simulink model "sampleModel7424_pp_difftest"  (R2018a)
settings: Solver=VariableStepAuto  StartTime=0.0  StopTime=10.0  RelTol=1e-3
undefined symbols (not defined in the file): DiscIntNeverNeededParam
libraries: simulink x211
(part 1 of 5)
settings Model: Creator=cyfuzz  LastModifiedBy=shafiul
settings CodeAppCC: StateflowObjectComments=on

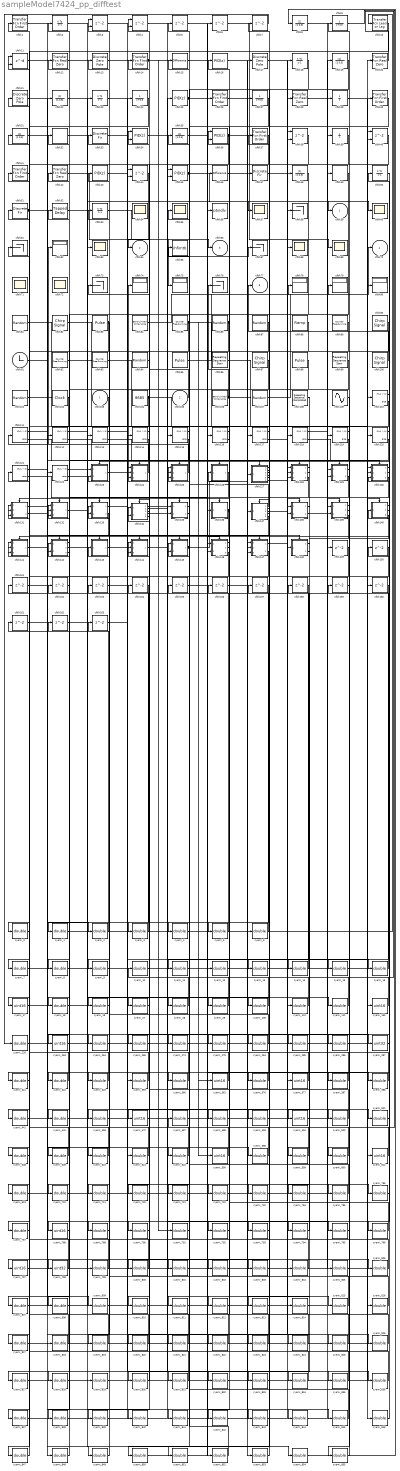
== system sampleModel7424_pp_difftest ==
  cfblk103 : Inport
  cfblk105 : Inport  Port=2
  cfblk{1,14,26,30,37,41} (6 alike) : simulink/Discrete/Transfer Fcn First Order  PoleZ=0.95  ICPrevOutput=0.0  DoSatur=off
      settings: SourceProductName=Simulink
  cfblk10 : simulink/Discrete/Transfer Fcn Lead or Lag  PoleZ=0.95  ZeroZ=0.75  ICPrevOutput=0.0  ICPrevInput=0.0  DoSatur=off
      settings: SourceProductName=Simulink  SourceProductBaseCode=SL
  cfblk{82,90,97,100} (4 alike) : simulink/Sources/Chirp Signal  f1=0.1  T=100  f2=1
  cfblk101 : UniformRandomNumber  SampleTime=0.1
  cfblk102 : DigitalClock
  cfblk104 : Constant  Value=8685  OutDataTypeStr=double  SampleTime=1
  cfblk106 : simulink/Sources/Band-Limited White Noise  Cov=[0.1]  Ts=0.1  seed=[23341]
  cfblk107 : RandomNumber  SampleTime=0.1
  cfblk108 : simulink/Sources/Repeating Sequence Interpolated  OutValues=[3 1 4 2 1].'  TimeValues=[0 0.1 0.5 0.6 1].'  LookUpMeth=Interpolation-Use End Values  tsamp=0.01  OutMin=[]  OutMax=[]  OutDataTypeStr=double  OutputDataTypeScalingMode=double  OutDataType=fixdt(0,8)  OutScaling=2^-10
  cfblk109 : Sin  SampleTime=0
  cfblk11 : Delay  DelayLengthSource=Input port  SampleTime=1
      settings: InputPortMap=u0,p1
  cfblk{110..122} (13 alike) : If  SampleTime=1
  cfblk{12,20,28,42} (4 alike) : simulink/Discrete/Transfer Fcn Real Zero  ZeroZ=0.75  ICPrevInput=0.0  DoSatur=off
      settings: SourceProductName=Simulink  SourceProductBaseCode=SL
  cfblk123 : Subsystem  TreatAsAtomicUnit=on
  cfblk124 : Subsystem  TreatAsAtomicUnit=on
  cfblk125 : Subsystem  TreatAsAtomicUnit=on
  cfblk126 : Subsystem  TreatAsAtomicUnit=on
  cfblk127 : Subsystem  TreatAsAtomicUnit=on
  cfblk128 : Subsystem  TreatAsAtomicUnit=on
  cfblk129 : Subsystem  TreatAsAtomicUnit=on
  cfblk13 : DiscreteZeroPole  Poles=[0 0.5]  Gain=1
  cfblk130 : Subsystem  TreatAsAtomicUnit=on
  cfblk131 : Subsystem  TreatAsAtomicUnit=on
  cfblk132 : Subsystem  TreatAsAtomicUnit=on
  cfblk133 : Subsystem  TreatAsAtomicUnit=on
  cfblk134 : Subsystem  TreatAsAtomicUnit=on
  cfblk135 : Subsystem  TreatAsAtomicUnit=on
  cfblk136 : Subsystem  TreatAsAtomicUnit=on
  cfblk137 : Subsystem  TreatAsAtomicUnit=on
  cfblk138 : Subsystem  TreatAsAtomicUnit=on
  cfblk139 : Subsystem  TreatAsAtomicUnit=on
  cfblk140 : Subsystem  TreatAsAtomicUnit=on
  cfblk141 : Subsystem  TreatAsAtomicUnit=on
  cfblk142 : Subsystem  TreatAsAtomicUnit=on
  cfblk143 : Subsystem  TreatAsAtomicUnit=on
  cfblk144 : Subsystem  TreatAsAtomicUnit=on
  cfblk145 : Subsystem  TreatAsAtomicUnit=on
  cfblk146 : Subsystem  TreatAsAtomicUnit=on
  cfblk147 : Subsystem  TreatAsAtomicUnit=on
  cfblk148 : Subsystem  TreatAsAtomicUnit=on
  cfblk{5..7,149..163} (18 alike) : Delay  SampleTime=1
  cfblk15 : simulink/Discrete/Difference  ICPrevInput=0.0  OutMin=[]  OutMax=[]  OutDataTypeStr=double  OutputDataTypeScalingMode=double  OutDataType=fixdt(1, 16)  OutScaling=2^-10  DoSatur=off
  cfblk16 : simulink/Continuous/PID Controller  Controller=PID  TimeDomain=Discrete-time  SampleTime=1  IntegratorMethod=Forward Euler  FilterMethod=Forward Euler  Form=Parallel  UseFilter=on  ControllerParametersSource=internal  P=1  I=1  D=0  N=100  InitialConditionSource=internal  InitialConditionForIntegrator=0  InitialConditionForFilter=0  ExternalReset=none  LimitOutput=off  UpperSaturationLimit=inf  LowerSaturationLimit=-inf  LinearizeAsGain=off  AntiWindupMode=none  Kb=1  TrackingMode=off  Kt=1  PParamMin=[]  PParamMax=[]  IParamMin=[]  IParamMax=[]  DParamMin=[]  DParamMax=[]  NParamMin=[]  NParamMax=[]  KbParamMin=[]  KbParamMax=[]  KtParamMin=[]  KtParamMax=[]  POutMin=[]  POutMax=[]  IOutMin=[]  IOutMax=[]  DOutMin=[]  DOutMax=[]  NOutMin=[]  NOutMax=[]  KbOutMin=[]  KbOutMax=[]  KtOutMin=[]  KtOutMax=[]  IntegratorOutMin=[]  IntegratorOutMax=[]  FilterOutMin=[]  FilterOutMax=[]  SumOutMin=[]  SumOutMax=[]  SumI1OutMin=[]  SumI1OutMax=[]  SumI2OutMin=[]  SumI2OutMax=[]  SumI3OutMin=[]  SumI3OutMax=[]  SumDOutMin=[]  SumDOutMax=[]  SaturationOutMin=[]  SaturationOutMax=[]  IntegratorContinuousStateAttributes=''  IntegratorStateMustResolveToSignalObject=off  IntegratorRTWStateStorageClass=Auto  FilterContinuousStateAttributes=''  FilterStateMustResolveToSignalObject=off  FilterRTWStateStorageClass=Auto  DifferentiatorICPrevScaledInput=0  DifferentiatorOutMin=[]  DifferentiatorOutMax=[]  FilterDiffOutCoefMin=[]  FilterDiffOutCoefMax=[]  SumDenOutMin=[]  SumDenOutMax=[]  SumNumOutMin=[]  SumNumOutMax=[]  ReciprocalOutMin=[]  ReciprocalOutMax=[]  DivideOutMin=[]  DivideOutMax=[]  TunerSelectOption=Transfer Function Based (PID Tuner App)
  cfblk17 : DiscreteZeroPole  Poles=[0 0.5]  Gain=1
  cfblk{2,18,23,50,53} (5 alike) : DiscreteIntegrator  OutDataTypeStr=double  ICPrevOutput=DiscIntNeverNeededParam  ICPrevScaledInput=DiscIntNeverNeededParam
  cfblk{8,19,22,31,35,48} (6 alike) : DiscreteFilter  SampleTime=1
  cfblk21 : DiscreteZeroPole  Poles=[0 0.5]  Gain=1
  cfblk24 : DiscreteTransferFcn  SampleTime=1
  cfblk25 : simulink/Continuous/PID Controller  Controller=PID  TimeDomain=Discrete-time  SampleTime=1  IntegratorMethod=Forward Euler  FilterMethod=Forward Euler  Form=Parallel  UseFilter=on  ControllerParametersSource=internal  P=1  I=1  D=0  N=100  InitialConditionSource=internal  InitialConditionForIntegrator=0  InitialConditionForFilter=0  ExternalReset=none  LimitOutput=off  UpperSaturationLimit=inf  LowerSaturationLimit=-inf  LinearizeAsGain=off  AntiWindupMode=none  Kb=1  TrackingMode=off  Kt=1  PParamMin=[]  PParamMax=[]  IParamMin=[]  IParamMax=[]  DParamMin=[]  DParamMax=[]  NParamMin=[]  NParamMax=[]  KbParamMin=[]  KbParamMax=[]  KtParamMin=[]  KtParamMax=[]  POutMin=[]  POutMax=[]  IOutMin=[]  IOutMax=[]  DOutMin=[]  DOutMax=[]  NOutMin=[]  NOutMax=[]  KbOutMin=[]  KbOutMax=[]  KtOutMin=[]  KtOutMax=[]  IntegratorOutMin=[]  IntegratorOutMax=[]  FilterOutMin=[]  FilterOutMax=[]  SumOutMin=[]  SumOutMax=[]  SumI1OutMin=[]  SumI1OutMax=[]  SumI2OutMin=[]  SumI2OutMax=[]  SumI3OutMin=[]  SumI3OutMax=[]  SumDOutMin=[]  SumDOutMax=[]  SaturationOutMin=[]  SaturationOutMax=[]  IntegratorContinuousStateAttributes=''  IntegratorStateMustResolveToSignalObject=off  IntegratorRTWStateStorageClass=Auto  FilterContinuousStateAttributes=''  FilterStateMustResolveToSignalObject=off  FilterRTWStateStorageClass=Auto  DifferentiatorICPrevScaledInput=0  DifferentiatorOutMin=[]  DifferentiatorOutMax=[]  FilterDiffOutCoefMin=[]  FilterDiffOutCoefMax=[]  SumDenOutMin=[]  SumDenOutMax=[]  SumNumOutMin=[]  SumNumOutMax=[]  ReciprocalOutMin=[]  ReciprocalOutMax=[]  DivideOutMin=[]  DivideOutMax=[]  TunerSelectOption=Transfer Function Based (PID Tuner App)
  cfblk27 : DiscreteTransferFcn  SampleTime=1
  cfblk29 : UnitDelay
  cfblk{3..4,38,40,44} (5 alike) : Delay  ShowEnablePort=on  SampleTime=1
      settings: InputPortMap=u0,e6
  cfblk32 : DiscreteStateSpace
  cfblk33 : DiscreteFir  SampleTime=1
  cfblk34 : simulink/Continuous/PID Controller (2DOF)  Controller=PID  TimeDomain=Discrete-time  SampleTime=1  IntegratorMethod=Forward Euler  FilterMethod=Forward Euler  Form=Parallel  UseFilter=on  ControllerParametersSource=internal  P=1  I=1  D=0  N=100  b=1  c=1  InitialConditionSource=internal  InitialConditionForIntegrator=0  InitialConditionForFilter=0  ExternalReset=none  LimitOutput=off  UpperSaturationLimit=inf  LowerSaturationLimit=-inf  LinearizeAsGain=off  AntiWindupMode=none  Kb=1  TrackingMode=off  Kt=1  PParamMin=[]  PParamMax=[]  IParamMin=[]  IParamMax=[]  DParamMin=[]  DParamMax=[]  NParamMin=[]  NParamMax=[]  bParamMin=[]  bParamMax=[]  cParamMin=[]  cParamMax=[]  KbParamMin=[]  KbParamMax=[]  KtParamMin=[]  KtParamMax=[]  POutMin=[]  POutMax=[]  IOutMin=[]  IOutMax=[]  DOutMin=[]  DOutMax=[]  NOutMin=[]  NOutMax=[]  bOutMin=[]  bOutMax=[]  cOutMin=[]  cOutMax=[]  KbOutMin=[]  KbOutMax=[]  KtOutMin=[]  KtOutMax=[]  IntegratorOutMin=[]  IntegratorOutMax=[]  FilterOutMin=[]  FilterOutMax=[]  SumOutMin=[]  SumOutMax=[]  Sum1OutMin=[]  Sum1OutMax=[]  Sum2OutMin=[]  Sum2OutMax=[]  Sum3OutMin=[]  Sum3OutMax=[]  SumI1OutMin=[]  SumI1OutMax=[]  SumI2OutMin=[]  SumI2OutMax=[]  SumI3OutMin=[]  SumI3OutMax=[]  SumDOutMin=[]  SumDOutMax=[]  SaturationOutMin=[]  SaturationOutMax=[]  IntegratorContinuousStateAttributes=''  IntegratorStateMustResolveToSignalObject=off  IntegratorRTWStateStorageClass=Auto  FilterContinuousStateAttributes=''  FilterStateMustResolveToSignalObject=off  FilterRTWStateStorageClass=Auto  DifferentiatorICPrevScaledInput=0  DifferentiatorOutMin=[]  DifferentiatorOutMax=[]  FilterDiffOutCoefMin=[]  FilterDiffOutCoefMax=[]  SumDenOutMin=[]  SumDenOutMax=[]  SumNumOutMin=[]  SumNumOutMax=[]  ReciprocalOutMin=[]  ReciprocalOutMax=[]  DivideOutMin=[]  DivideOutMax=[]  TunerSelectOption=Transfer Function Based (PID Tuner App)
  cfblk36 : simulink/Continuous/PID Controller (2DOF)  Controller=PID  TimeDomain=Discrete-time  SampleTime=1  IntegratorMethod=Forward Euler  FilterMethod=Forward Euler  Form=Parallel  UseFilter=on  ControllerParametersSource=internal  P=1  I=1  D=0  N=100  b=1  c=1  InitialConditionSource=internal  InitialConditionForIntegrator=0  InitialConditionForFilter=0  ExternalReset=none  LimitOutput=off  UpperSaturationLimit=inf  LowerSaturationLimit=-inf  LinearizeAsGain=off  AntiWindupMode=none  Kb=1  TrackingMode=off  Kt=1  PParamMin=[]  PParamMax=[]  IParamMin=[]  IParamMax=[]  DParamMin=[]  DParamMax=[]  NParamMin=[]  NParamMax=[]  bParamMin=[]  bParamMax=[]  cParamMin=[]  cParamMax=[]  KbParamMin=[]  KbParamMax=[]  KtParamMin=[]  KtParamMax=[]  POutMin=[]  POutMax=[]  IOutMin=[]  IOutMax=[]  DOutMin=[]  DOutMax=[]  NOutMin=[]  NOutMax=[]  bOutMin=[]  bOutMax=[]  cOutMin=[]  cOutMax=[]  KbOutMin=[]  KbOutMax=[]  KtOutMin=[]  KtOutMax=[]  IntegratorOutMin=[]  IntegratorOutMax=[]  FilterOutMin=[]  FilterOutMax=[]  SumOutMin=[]  SumOutMax=[]  Sum1OutMin=[]  Sum1OutMax=[]  Sum2OutMin=[]  Sum2OutMax=[]  Sum3OutMin=[]  Sum3OutMax=[]  SumI1OutMin=[]  SumI1OutMax=[]  SumI2OutMin=[]  SumI2OutMax=[]  SumI3OutMin=[]  SumI3OutMax=[]  SumDOutMin=[]  SumDOutMax=[]  SaturationOutMin=[]  SaturationOutMax=[]  IntegratorContinuousStateAttributes=''  IntegratorStateMustResolveToSignalObject=off  IntegratorRTWStateStorageClass=Auto  FilterContinuousStateAttributes=''  FilterStateMustResolveToSignalObject=off  FilterRTWStateStorageClass=Auto  DifferentiatorICPrevScaledInput=0  DifferentiatorOutMin=[]  DifferentiatorOutMax=[]  FilterDiffOutCoefMin=[]  FilterDiffOutCoefMax=[]  SumDenOutMin=[]  SumDenOutMax=[]  SumNumOutMin=[]  SumNumOutMax=[]  ReciprocalOutMin=[]  ReciprocalOutMax=[]  DivideOutMin=[]  DivideOutMax=[]  TunerSelectOption=Transfer Function Based (PID Tuner App)
  cfblk39 : UnitDelay
  cfblk43 : simulink/Continuous/PID Controller  Controller=PID  TimeDomain=Discrete-time  SampleTime=1  IntegratorMethod=Forward Euler  FilterMethod=Forward Euler  Form=Parallel  UseFilter=on  ControllerParametersSource=internal  P=1  I=1  D=0  N=100  InitialConditionSource=internal  InitialConditionForIntegrator=0  InitialConditionForFilter=0  ExternalReset=none  LimitOutput=off  UpperSaturationLimit=inf  LowerSaturationLimit=-inf  LinearizeAsGain=off  AntiWindupMode=none  Kb=1  TrackingMode=off  Kt=1  PParamMin=[]  PParamMax=[]  IParamMin=[]  IParamMax=[]  DParamMin=[]  DParamMax=[]  NParamMin=[]  NParamMax=[]  KbParamMin=[]  KbParamMax=[]  KtParamMin=[]  KtParamMax=[]  POutMin=[]  POutMax=[]  IOutMin=[]  IOutMax=[]  DOutMin=[]  DOutMax=[]  NOutMin=[]  NOutMax=[]  KbOutMin=[]  KbOutMax=[]  KtOutMin=[]  KtOutMax=[]  IntegratorOutMin=[]  IntegratorOutMax=[]  FilterOutMin=[]  FilterOutMax=[]  SumOutMin=[]  SumOutMax=[]  SumI1OutMin=[]  SumI1OutMax=[]  SumI2OutMin=[]  SumI2OutMax=[]  SumI3OutMin=[]  SumI3OutMax=[]  SumDOutMin=[]  SumDOutMax=[]  SaturationOutMin=[]  SaturationOutMax=[]  IntegratorContinuousStateAttributes=''  IntegratorStateMustResolveToSignalObject=off  IntegratorRTWStateStorageClass=Auto  FilterContinuousStateAttributes=''  FilterStateMustResolveToSignalObject=off  FilterRTWStateStorageClass=Auto  DifferentiatorICPrevScaledInput=0  DifferentiatorOutMin=[]  DifferentiatorOutMax=[]  FilterDiffOutCoefMin=[]  FilterDiffOutCoefMax=[]  SumDenOutMin=[]  SumDenOutMax=[]  SumNumOutMin=[]  SumNumOutMax=[]  ReciprocalOutMin=[]  ReciprocalOutMax=[]  DivideOutMin=[]  DivideOutMax=[]  TunerSelectOption=Transfer Function Based (PID Tuner App)
  cfblk45 : simulink/Continuous/PID Controller (2DOF)  Controller=PID  TimeDomain=Discrete-time  SampleTime=1  IntegratorMethod=Forward Euler  FilterMethod=Forward Euler  Form=Parallel  UseFilter=on  ControllerParametersSource=internal  P=1  I=1  D=0  N=100  b=1  c=1  InitialConditionSource=internal  InitialConditionForIntegrator=0  InitialConditionForFilter=0  ExternalReset=none  LimitOutput=off  UpperSaturationLimit=inf  LowerSaturationLimit=-inf  LinearizeAsGain=off  AntiWindupMode=none  Kb=1  TrackingMode=off  Kt=1  PParamMin=[]  PParamMax=[]  IParamMin=[]  IParamMax=[]  DParamMin=[]  DParamMax=[]  NParamMin=[]  NParamMax=[]  bParamMin=[]  bParamMax=[]  cParamMin=[]  cParamMax=[]  KbParamMin=[]  KbParamMax=[]  KtParamMin=[]  KtParamMax=[]  POutMin=[]  POutMax=[]  IOutMin=[]  IOutMax=[]  DOutMin=[]  DOutMax=[]  NOutMin=[]  NOutMax=[]  bOutMin=[]  bOutMax=[]  cOutMin=[]  cOutMax=[]  KbOutMin=[]  KbOutMax=[]  KtOutMin=[]  KtOutMax=[]  IntegratorOutMin=[]  IntegratorOutMax=[]  FilterOutMin=[]  FilterOutMax=[]  SumOutMin=[]  SumOutMax=[]  Sum1OutMin=[]  Sum1OutMax=[]  Sum2OutMin=[]  Sum2OutMax=[]  Sum3OutMin=[]  Sum3OutMax=[]  SumI1OutMin=[]  SumI1OutMax=[]  SumI2OutMin=[]  SumI2OutMax=[]  SumI3OutMin=[]  SumI3OutMax=[]  SumDOutMin=[]  SumDOutMax=[]  SaturationOutMin=[]  SaturationOutMax=[]  IntegratorContinuousStateAttributes=''  IntegratorStateMustResolveToSignalObject=off  IntegratorRTWStateStorageClass=Auto  FilterContinuousStateAttributes=''  FilterStateMustResolveToSignalObject=off  FilterRTWStateStorageClass=Auto  DifferentiatorICPrevScaledInput=0  DifferentiatorOutMin=[]  DifferentiatorOutMax=[]  FilterDiffOutCoefMin=[]  FilterDiffOutCoefMax=[]  SumDenOutMin=[]  SumDenOutMax=[]  SumNumOutMin=[]  SumNumOutMax=[]  ReciprocalOutMin=[]  ReciprocalOutMax=[]  DivideOutMin=[]  DivideOutMax=[]  TunerSelectOption=Transfer Function Based (PID Tuner App)
  cfblk46 : simulink/Discrete/Difference  ICPrevInput=0.0  OutMin=[]  OutMax=[]  OutDataTypeStr=double  OutputDataTypeScalingMode=double  OutDataType=fixdt(1, 16)  OutScaling=2^-10  DoSatur=off
  cfblk47 : DiscreteFir  SampleTime=1
  cfblk49 : DiscreteStateSpace
  cfblk51 : DiscreteFir  SampleTime=1
  cfblk52 : simulink/Discrete/Tapped Delay  vinit=0.0  samptime=-1  NumDelays=1  DelayOrder=Oldest  includeCurrent=off
  cfblk{54..55,57,60,63,68..69,71..72} (9 alike) : Scope
      cfblk54 settings: Floating=on
      cfblk71 settings: Floating=on
      cfblk72 settings: Floating=on
  cfblk56 : ToWorkspace  VariableName=ptxidlv  SaveFormat=Timeseries  SampleTime=-1
  cfblk{58,61,67,73,76} (5 alike) : Terminator
  cfblk{62,74..75,78..80} (6 alike) : Display
  cfblk65 : ToWorkspace  VariableName=ihfimtb  SaveFormat=Timeseries  SampleTime=-1
  cfblk81 : RandomNumber  SampleTime=0.1
  cfblk83 : DiscretePulseGenerator  PulseType=Time based  Period=10  PulseWidth=5
  cfblk84 : simulink/Sources/Band-Limited White Noise  Cov=[0.1]  Ts=0.1  seed=[23341]
  cfblk{85,89,92..93} (4 alike) : simulink/Sources/Counter Free-Running  NumBits=16  tsamp=1
  cfblk86 : UniformRandomNumber  SampleTime=0.1
  cfblk87 : RandomNumber  SampleTime=0.1
  cfblk88 : simulink/Sources/Ramp  slope=1  start=0  InitialOutput=0
  cfblk9 : DiscreteTransferFcn  SampleTime=1
  cfblk91 : Clock
  cfblk94 : UniformRandomNumber  SampleTime=0.1
  cfblk95 : DiscretePulseGenerator  PulseType=Time based  Period=10  PulseWidth=5
  cfblk96 : simulink/Sources/Repeating Sequence Stair  OutValues=[3 1 4 2 1].'  tsamp=1  OutMin=[]  OutMax=[]  OutDataTypeStr=double  OutputDataTypeScalingMode=double  OutDataType=fixdt(0,8)  ConRadixGroup=Best Precision: Vector-wise  OutScaling=2^-12
  cfblk98 : DiscretePulseGenerator  PulseType=Time based  Period=10  PulseWidth=5
  cfblk99 : simulink/Sources/Repeating Sequence Stair  OutValues=[3 1 4 2 1].'  tsamp=1  OutMin=[]  OutMax=[]  OutDataTypeStr=double  OutputDataTypeScalingMode=double  OutDataType=fixdt(0,8)  ConRadixGroup=Best Precision: Vector-wise  OutScaling=2^-12
  cyemi_{0..16,18..19,27..29,109..111,226,264..265,274..275,284..286,321..323,359..360,376,397..398,441..442,458,487..488,493,500..501,508..510,521..522,598..600,613,710..711,720..722,732,784..787,789..796,799..855} (133 alike) : DataTypeConversion  OutDataTypeStr=double
  cyemi_{17,153,263,361,377,472,494,590,612,788,797} (11 alike) : DataTypeConversion  OutDataTypeStr=uint16
  cyemi_287 : DataTypeConversion  OutDataTypeStr=uint32
  cyemi_798 : DataTypeConversion  OutDataTypeStr=uint32
  cfblk59 : Outport
  cfblk64 : Outport  Port=2
  cfblk66 : Outport  Port=3
  cfblk70 : Outport  Port=4
  cfblk77 : Outport  Port=5
  wires:
  cfblk100/1 -> cfblk77/1
  cfblk105/1 -> cfblk73/1
  cfblk42/1 -> cfblk66/1
  cfblk83/1 -> cyemi_9/1, cyemi_710/1
  cfblk84/1 -> cfblk78/1
  cfblk45/1 -> cfblk59/1, cyemi_845/1
  cfblk95/1 -> cfblk70/1
  cfblk6/1 -> cfblk69/1
  cfblk25/1 -> cyemi_732/1, cyemi_851/1
  cfblk132/1(cfblk2) -> cfblk63/1
  cfblk14/1 -> cyemi_15/1, cyemi_791/1
  cfblk17/1 -> cfblk58/1
  cfblk53/1 -> cfblk75/1
  cfblk136/1(cfblk2) -> cyemi_0/1, cyemi_711/1
  cfblk124/1(cfblk2) -> cfblk61/1
  cfblk137/1(cfblk2) -> cfblk55/1
  cfblk123/1(cfblk2) -> cfblk74/1
  cfblk44/1 -> cfblk64/1
  cfblk145/1(cfblk2) -> cfblk79/1, cyemi_361/1
  cfblk86/1 -> cyemi_510/1, cyemi_819/1
  cfblk51/1 -> cyemi_2/1, cyemi_843/1
  cfblk2/1 -> cfblk57/1
  cfblk28/1 -> cfblk60/1
  cfblk106/1 -> cfblk76/1, cyemi_110/1
  cfblk107/1 -> cfblk80/1
  cfblk104/1 -> cyemi_6/1, cyemi_441/1
  cfblk36/1 -> cyemi_28/1, cyemi_111/1
  cfblk85/1 -> cyemi_377/1, cyemi_472/1, cyemi_590/1
  cfblk134/4(cfblk16) -> cfblk67/1
  cfblk125/1(cfblk2) -> cfblk62/1
  cfblk127/6(cfblk17) -> cfblk68/1
  cfblk110/1 -> cfblk123/Action
  cfblk110/2 -> cfblk124/Action
  cfblk111/1 -> cfblk125/Action
  cfblk111/2 -> cfblk126/Action
  cfblk112/1 -> cfblk127/Action
  cfblk112/2 -> cfblk128/Action
  cfblk113/1 -> cfblk129/Action
  cfblk113/2 -> cfblk130/Action
  cfblk114/1 -> cfblk131/Action
  cfblk114/2 -> cfblk132/Action
  cfblk115/1 -> cfblk133/Action
  cfblk115/2 -> cfblk134/Action
  cfblk116/1 -> cfblk135/Action
  cfblk116/2 -> cfblk136/Action
  cfblk117/1 -> cfblk137/Action
  cfblk117/2 -> cfblk138/Action
  cfblk118/1 -> cfblk139/Action
  cfblk118/2 -> cfblk140/Action
  cfblk119/1 -> cfblk141/Action
  cfblk119/2 -> cfblk142/Action
  cfblk120/1 -> cfblk143/Action
  cfblk120/2 -> cfblk144/Action
  cfblk121/1 -> cfblk145/Action
  cfblk121/2 -> cfblk146/Action
  cfblk122/1 -> cfblk147/Action
  cfblk122/2 -> cfblk148/Action
  cyemi_0/1 -> cfblk1/1
  cyemi_1/1 -> cfblk10/1
  cfblk127/3(cfblk14) -> cyemi_1/1
  cyemi_2/1 -> cfblk11/1
  cyemi_3/1 -> cfblk11/2
  cfblk127/1(cfblk2) -> cyemi_3/1
  cyemi_4/1 -> cfblk110/1
  cfblk135/2(cfblk14) -> cyemi_4/1
  cyemi_5/1 -> cfblk111/1
  cfblk87/1 -> cyemi_5/1
  cyemi_6/1 -> cfblk112/1
  cyemi_7/1 -> cfblk113/1
  cfblk24/1 -> cyemi_7/1
  cyemi_8/1 -> cfblk114/1
  cfblk157/1 -> cyemi_8/1
  cyemi_9/1 -> cfblk115/1
  cyemi_10/1 -> cfblk116/1
  cfblk20/1 -> cyemi_10/1
  cyemi_11/1 -> cfblk117/1
  cfblk129/2(cfblk9) -> cyemi_11/1
  cyemi_12/1 -> cfblk118/1
  cfblk155/1 -> cyemi_12/1
  cyemi_13/1 -> cfblk119/1
  cfblk138/1(cfblk2) -> cyemi_13/1
  cyemi_14/1 -> cfblk12/1
  cfblk33/1 -> cyemi_14/1
  cyemi_15/1 -> cfblk120/1
  cyemi_16/1 -> cfblk121/1
  cfblk8/1 -> cyemi_16/1
  cyemi_17/1 -> cfblk122/1
  cfblk89/1 -> cyemi_17/1
  cyemi_18/1 -> cfblk123/1(cfblk1)
  cfblk103/1 -> cyemi_18/1
  cyemi_19/1 -> cfblk123/2(cfblk10)
  cfblk127/2(cfblk13) -> cyemi_19/1
  cyemi_27/1 -> cfblk124/1(cfblk1)
  cfblk135/1(cfblk2) -> cyemi_27/1
  cyemi_28/1 -> cfblk124/2(cfblk12)
  cyemi_29/1 -> cfblk124/3(cfblk13)
  cfblk128/3(cfblk12) -> cyemi_29/1
  cyemi_109/1 -> cfblk125/1(cfblk1)
  cfblk22/1 -> cyemi_109/1
  cyemi_110/1 -> cfblk125/2(cfblk9)
  cyemi_111/1 -> cfblk125/3(cfblk10)
  cyemi_153/1 -> cfblk126/1(cfblk1)
  cfblk93/1 -> cyemi_153/1
  cyemi_226/1 -> cfblk127/1(cfblk1)
  cfblk7/1 -> cyemi_226/1
  cyemi_263/1 -> cfblk128/1(cfblk1)
  cfblk152/1 -> cyemi_263/1
  cyemi_264/1 -> cfblk128/2(cfblk9)
  cfblk151/1 -> cyemi_264/1
  cyemi_265/1 -> cfblk128/3(cfblk10)
  cfblk130/1(cfblk2) -> cyemi_265/1
  cyemi_274/1 -> cfblk129/1(cfblk1)
  cfblk162/1 -> cyemi_274/1
  cyemi_275/1 -> cfblk129/2(cfblk8)
  cfblk27/1 -> cyemi_275/1
  cyemi_284/1 -> cfblk13/1
  cfblk38/1 -> cyemi_284/1
  cyemi_285/1 -> cfblk130/1(cfblk1)
  cfblk108/1 -> cyemi_285/1
  cyemi_286/1 -> cfblk130/2(cfblk7)
  cfblk129/1(cfblk2) -> cyemi_286/1
  cyemi_287/1 -> cfblk130/3(cfblk8)
  cfblk161/1 -> cyemi_287/1
  cyemi_321/1 -> cfblk131/1(cfblk1)
  cfblk150/1 -> cyemi_321/1
  cyemi_322/1 -> cfblk131/2(cfblk13)
  cfblk140/1(cfblk2) -> cyemi_322/1
  cyemi_323/1 -> cfblk131/3(cfblk14)
  cfblk154/1 -> cyemi_323/1
  cyemi_359/1 -> cfblk132/1(cfblk1)
  cfblk163/1 -> cyemi_359/1
  cyemi_360/1 -> cfblk132/2(cfblk13)
  cfblk140/2(cfblk7) -> cyemi_360/1
  cyemi_361/1 -> cfblk132/3(cfblk14)
  cyemi_376/1 -> cfblk133/1(cfblk1)
  cfblk15/1 -> cyemi_376/1
  cyemi_377/1 -> cfblk133/2(cfblk16)
  cyemi_397/1 -> cfblk134/1(cfblk1)
  cfblk159/1 -> cyemi_397/1
  cyemi_398/1 -> cfblk134/2(cfblk13)
  cfblk156/1 -> cyemi_398/1
  cyemi_441/1 -> cfblk135/1(cfblk1)
  cyemi_442/1 -> cfblk135/2(cfblk13)
  cfblk142/3(cfblk15) -> cyemi_442/1
  cyemi_458/1 -> cfblk136/1(cfblk1)
  cfblk127/5(cfblk16) -> cyemi_458/1
  cyemi_472/1 -> cfblk137/1(cfblk1)
  cyemi_487/1 -> cfblk138/1(cfblk1)
  cfblk9/1 -> cyemi_487/1
  cyemi_488/1 -> cfblk138/2(cfblk6)
  cfblk97/1 -> cyemi_488/1
  cyemi_493/1 -> cfblk139/1(cfblk1)
  cfblk88/1 -> cyemi_493/1
  cyemi_494/1 -> cfblk139/2(cfblk8)
  cfblk160/1 -> cyemi_494/1
  cyemi_500/1 -> cfblk14/1
  cfblk13/1 -> cyemi_500/1
  cyemi_501/1 -> cfblk140/1(cfblk1)
  cfblk133/1(cfblk2) -> cyemi_501/1
  cyemi_508/1 -> cfblk141/1(cfblk1)
  cfblk10/1 -> cyemi_508/1
  cyemi_509/1 -> cfblk141/2(cfblk13)
  cfblk99/1 -> cyemi_509/1
  cyemi_510/1 -> cfblk141/3(cfblk14)
  cyemi_521/1 -> cfblk142/1(cfblk1)
  cfblk3/1 -> cyemi_521/1
  cyemi_522/1 -> cfblk142/2(cfblk13)
  cfblk131/2(cfblk15) -> cyemi_522/1
  cyemi_590/1 -> cfblk143/1(cfblk1)
  cyemi_598/1 -> cfblk144/1(cfblk1)
  cfblk31/1 -> cyemi_598/1
  cyemi_599/1 -> cfblk144/2(cfblk12)
  cfblk148/2(cfblk17) -> cyemi_599/1
  cyemi_600/1 -> cfblk144/3(cfblk13)
  cfblk130/3(cfblk10) -> cyemi_600/1
  cyemi_612/1 -> cfblk145/1(cfblk1)
  cfblk92/1 -> cyemi_612/1
  cyemi_613/1 -> cfblk145/2(cfblk16)
  cfblk39/1 -> cyemi_613/1
  cyemi_710/1 -> cfblk146/1(cfblk1)
  cyemi_711/1 -> cfblk146/2(cfblk10)
  cyemi_720/1 -> cfblk147/1(cfblk1)
  cfblk40/1 -> cyemi_720/1
  cyemi_721/1 -> cfblk147/2(cfblk10)
  cfblk37/1 -> cyemi_721/1
  cyemi_722/1 -> cfblk147/3(cfblk11)
  cfblk153/1 -> cyemi_722/1
  cyemi_732/1 -> cfblk148/1(cfblk1)
  cyemi_784/1 -> cfblk149/1
  cfblk128/1(cfblk2) -> cyemi_784/1
  cyemi_785/1 -> cfblk15/1
  cfblk147/1(cfblk2) -> cyemi_785/1
  cyemi_786/1 -> cfblk150/1
  cfblk143/1(cfblk2) -> cyemi_786/1
  cyemi_787/1 -> cfblk151/1
  cfblk41/1 -> cyemi_787/1
  cyemi_788/1 -> cfblk152/1
  cfblk139/1(cfblk2) -> cyemi_788/1
  cyemi_789/1 -> cfblk153/1
  cfblk139/2(cfblk9) -> cyemi_789/1
  cyemi_790/1 -> cfblk154/1
  cfblk139/3(cfblk10) -> cyemi_790/1
  cyemi_791/1 -> cfblk155/1
  cyemi_792/1 -> cfblk156/1
  cfblk130/2(cfblk9) -> cyemi_792/1
  cyemi_793/1 -> cfblk157/1
  cfblk34/1 -> cyemi_793/1
  cyemi_794/1 -> cfblk158/1
  cfblk35/1 -> cyemi_794/1
  cyemi_795/1 -> cfblk159/1
  cfblk137/3(cfblk12) -> cyemi_795/1
  cyemi_796/1 -> cfblk16/1
  cfblk50/1 -> cyemi_796/1
  cyemi_797/1 -> cfblk160/1
  cfblk137/4(cfblk13) -> cyemi_797/1
  cyemi_798/1 -> cfblk161/1
  cfblk137/5(cfblk14) -> cyemi_798/1
  cyemi_799/1 -> cfblk162/1
  cfblk52/1 -> cyemi_799/1
  cyemi_800/1 -> cfblk163/1
  cfblk146/2(cfblk11) -> cyemi_800/1
  cyemi_801/1 -> cfblk17/1
  cfblk30/1 -> cyemi_801/1
  cyemi_802/1 -> cfblk18/1
  cfblk23/1 -> cyemi_802/1
  cyemi_803/1 -> cfblk19/1
  cfblk4/1 -> cyemi_803/1
  cyemi_804/1 -> cfblk2/1
  cfblk81/1 -> cyemi_804/1
  cyemi_805/1 -> cfblk20/1
  cfblk138/2(cfblk7) -> cyemi_805/1
  cyemi_806/1 -> cfblk21/1
  cfblk26/1 -> cyemi_806/1
  cyemi_807/1 -> cfblk22/1
  cfblk142/1(cfblk2) -> cyemi_807/1
  cyemi_808/1 -> cfblk23/1
  cfblk126/1(cfblk2) -> cyemi_808/1
  cyemi_809/1 -> cfblk24/1
  cfblk131/1(cfblk2) -> cyemi_809/1
  cyemi_810/1 -> cfblk25/1
  cfblk94/1 -> cyemi_810/1
  cyemi_811/1 -> cfblk26/1
  cfblk146/1(cfblk2) -> cyemi_811/1
  cyemi_812/1 -> cfblk27/1
  cfblk148/1(cfblk2) -> cyemi_812/1
  cyemi_813/1 -> cfblk28/1
  cfblk90/1 -> cyemi_813/1
  cyemi_814/1 -> cfblk29/1
  cfblk96/1 -> cyemi_814/1
  cyemi_815/1 -> cfblk3/1
  cfblk46/1 -> cyemi_815/1
  cyemi_816/1 -> cfblk3/2
  cfblk82/1 -> cyemi_816/1
  cyemi_817/1 -> cfblk30/1
  cfblk146/3(cfblk12) -> cyemi_817/1
  cyemi_818/1 -> cfblk31/1
  cfblk91/1 -> cyemi_818/1
  cyemi_819/1 -> cfblk32/1
  cyemi_820/1 -> cfblk33/1
  cfblk140/3(cfblk8) -> cyemi_820/1
  cyemi_821/1 -> cfblk34/1
  cfblk18/1 -> cyemi_821/1
  cyemi_822/1 -> cfblk34/2
  cfblk134/2(cfblk14) -> cyemi_822/1
  cyemi_823/1 -> cfblk35/1
  cfblk137/2(cfblk11) -> cyemi_823/1
  cyemi_824/1 -> cfblk36/1
  cfblk141/1(cfblk2) -> cyemi_824/1
  cyemi_825/1 -> cfblk36/2
  cfblk16/1 -> cyemi_825/1
  cyemi_826/1 -> cfblk37/1
  cfblk47/1 -> cyemi_826/1
  cyemi_827/1 -> cfblk38/1
  cfblk128/2(cfblk11) -> cyemi_827/1
  cyemi_828/1 -> cfblk38/2
  cfblk133/2(cfblk17) -> cyemi_828/1
  cyemi_829/1 -> cfblk39/1
  cfblk142/2(cfblk14) -> cyemi_829/1
  cyemi_830/1 -> cfblk4/1
  cfblk48/1 -> cyemi_830/1
  cyemi_831/1 -> cfblk4/2
  cfblk158/1 -> cyemi_831/1
  cyemi_832/1 -> cfblk40/1
  cfblk149/1 -> cyemi_832/1
  cyemi_833/1 -> cfblk40/2
  cfblk19/1 -> cyemi_833/1
  cyemi_834/1 -> cfblk41/1
  cfblk144/1(cfblk2) -> cyemi_834/1
  cyemi_835/1 -> cfblk42/1
  cfblk43/1 -> cyemi_835/1
  cyemi_836/1 -> cfblk43/1
  cfblk134/1(cfblk2) -> cyemi_836/1
  cyemi_837/1 -> cfblk44/1
  cfblk147/2(cfblk12) -> cyemi_837/1
  cyemi_838/1 -> cfblk44/2
  cfblk49/1 -> cyemi_838/1
  cyemi_839/1 -> cfblk45/1
  cfblk134/3(cfblk15) -> cyemi_839/1
  cyemi_840/1 -> cfblk45/2
  cfblk134/5(cfblk17) -> cyemi_840/1
  cyemi_841/1 -> cfblk46/1
  cfblk1/1 -> cyemi_841/1
  cyemi_842/1 -> cfblk47/1
  cfblk98/1 -> cyemi_842/1
  cyemi_843/1 -> cfblk48/1
  cyemi_844/1 -> cfblk49/1
  cfblk32/1 -> cyemi_844/1
  cyemi_845/1 -> cfblk5/1
  cyemi_846/1 -> cfblk50/1
  cfblk29/1 -> cyemi_846/1
  cyemi_847/1 -> cfblk51/1
  cfblk102/1 -> cyemi_847/1
  cyemi_848/1 -> cfblk52/1
  cfblk21/1 -> cyemi_848/1
  cyemi_849/1 -> cfblk53/1
  cfblk11/1 -> cyemi_849/1
  cyemi_850/1 -> cfblk56/1
  cfblk127/4(cfblk15) -> cyemi_850/1
  cyemi_851/1 -> cfblk6/1
  cyemi_852/1 -> cfblk65/1
  cfblk5/1 -> cyemi_852/1
  cyemi_853/1 -> cfblk7/1
  cfblk101/1 -> cyemi_853/1
  cyemi_854/1 -> cfblk8/1
  cfblk12/1 -> cyemi_854/1
  cyemi_855/1 -> cfblk9/1
  cfblk109/1 -> cyemi_855/1

== system sampleModel7424_pp_difftest/cfblk123 ==
  cfblk1 : Inport
  cfblk10 : Inport  Port=2
  Action Port : ActionPort  ActionType=then
  cfblk3 : UnitDelay  SampleTime=-1
  cfblk4 : simulink/Continuous/PID Controller  Controller=PID  TimeDomain=Discrete-time  SampleTime=-1  IntegratorMethod=Forward Euler  FilterMethod=Forward Euler  Form=Parallel  UseFilter=on  ControllerParametersSource=internal  P=1  I=1  D=0  N=100  InitialConditionSource=internal  InitialConditionForIntegrator=0  InitialConditionForFilter=0  ExternalReset=none  LimitOutput=off  UpperSaturationLimit=inf  LowerSaturationLimit=-inf  LinearizeAsGain=off  AntiWindupMode=none  Kb=1  TrackingMode=off  Kt=1  PParamMin=[]  PParamMax=[]  IParamMin=[]  IParamMax=[]  DParamMin=[]  DParamMax=[]  NParamMin=[]  NParamMax=[]  KbParamMin=[]  KbParamMax=[]  KtParamMin=[]  KtParamMax=[]  POutMin=[]  POutMax=[]  IOutMin=[]  IOutMax=[]  DOutMin=[]  DOutMax=[]  NOutMin=[]  NOutMax=[]  KbOutMin=[]  KbOutMax=[]  KtOutMin=[]  KtOutMax=[]  IntegratorOutMin=[]  IntegratorOutMax=[]  FilterOutMin=[]  FilterOutMax=[]  SumOutMin=[]  SumOutMax=[]  SumI1OutMin=[]  SumI1OutMax=[]  SumI2OutMin=[]  SumI2OutMax=[]  SumI3OutMin=[]  SumI3OutMax=[]  SumDOutMin=[]  SumDOutMax=[]  SaturationOutMin=[]  SaturationOutMax=[]  IntegratorContinuousStateAttributes=''  IntegratorStateMustResolveToSignalObject=off  IntegratorRTWStateStorageClass=Auto  FilterContinuousStateAttributes=''  FilterStateMustResolveToSignalObject=off  FilterRTWStateStorageClass=Auto  DifferentiatorICPrevScaledInput=0  DifferentiatorOutMin=[]  DifferentiatorOutMax=[]  FilterDiffOutCoefMin=[]  FilterDiffOutCoefMax=[]  SumDenOutMin=[]  SumDenOutMax=[]  SumNumOutMin=[]  SumNumOutMax=[]  ReciprocalOutMin=[]  ReciprocalOutMax=[]  DivideOutMin=[]  DivideOutMax=[]  TunerSelectOption=Transfer Function Based (PID Tuner App)
  cfblk5 : DiscreteTransferFcn
  cfblk6 : DiscreteIntegrator  SampleTime=-1  OutDataTypeStr=double  ICPrevOutput=DiscIntNeverNeededParam  ICPrevScaledInput=DiscIntNeverNeededParam
  cfblk7 : Delay
  cfblk8 : simulink/Discrete/Tapped Delay  vinit=0.0  samptime=-1  NumDelays=1  DelayOrder=Oldest  includeCurrent=off
  cfblk9 : DiscreteTransferFcn
  cyemi_{20..26} (7 alike) : DataTypeConversion  OutDataTypeStr=double
  cfblk2 : Outport
  wires:
  cfblk9/1 -> cfblk2/1
  cyemi_20/1 -> cfblk3/1
  cfblk7/1 -> cyemi_20/1
  cyemi_21/1 -> cfblk4/1
  cfblk10/1 -> cyemi_21/1
  cyemi_22/1 -> cfblk5/1
  cfblk3/1 -> cyemi_22/1
  cyemi_23/1 -> cfblk6/1
  cfblk8/1 -> cyemi_23/1
  cyemi_24/1 -> cfblk7/1
  cfblk6/1 -> cyemi_24/1
  cyemi_25/1 -> cfblk8/1
  cfblk4/1 -> cyemi_25/1
  cyemi_26/1 -> cfblk9/1
  cfblk1/1 -> cyemi_26/1

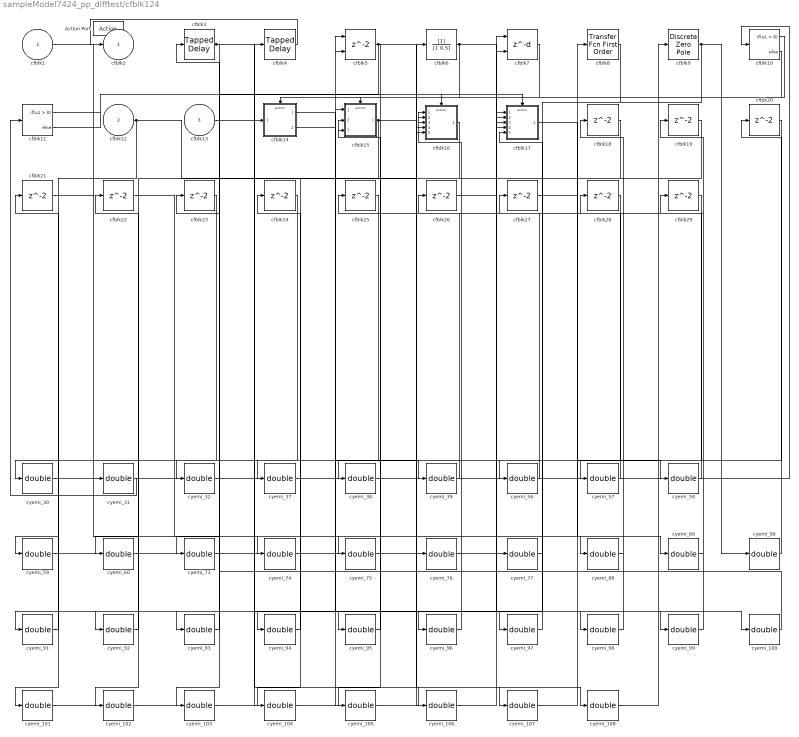
== system sampleModel7424_pp_difftest/cfblk124 ==
  cfblk1 : Inport
  cfblk12 : Inport  Port=2
  cfblk13 : Inport  Port=3
  Action Port : ActionPort  ActionType=else
  cfblk10 : If  SampleTime=1
  cfblk11 : If  SampleTime=1
  cfblk14 : Subsystem  TreatAsAtomicUnit=on
  cfblk15 : Subsystem  TreatAsAtomicUnit=on
  cfblk16 : Subsystem  TreatAsAtomicUnit=on
  cfblk17 : Subsystem  TreatAsAtomicUnit=on
  cfblk{18..29} (12 alike) : Delay
  cfblk3 : simulink/Discrete/Tapped Delay  vinit=0.0  samptime=-1  NumDelays=1  DelayOrder=Oldest  includeCurrent=off
  cfblk4 : simulink/Discrete/Tapped Delay  vinit=0.0  samptime=-1  NumDelays=1  DelayOrder=Oldest  includeCurrent=off
  cfblk5 : Delay  ShowEnablePort=on
      settings: InputPortMap=u0,e6
  cfblk6 : DiscreteFilter
  cfblk7 : Delay  DelayLengthSource=Input port
      settings: InputPortMap=u0,p1
  cfblk8 : simulink/Discrete/Transfer Fcn First Order  PoleZ=0.95  ICPrevOutput=0.0  DoSatur=off
      settings: SourceProductName=Simulink
  cfblk9 : DiscreteZeroPole  Poles=[0 0.5]  Gain=1  SampleTime=-1
  cyemi_{30..32,37..39,56..60,73..77,88..108} (37 alike) : DataTypeConversion  OutDataTypeStr=double
  cfblk2 : Outport
  wires:
  cfblk15/1(cfblk2) -> cyemi_97/1, cyemi_100/1, cyemi_102/1
  cfblk5/1 -> cyemi_93/1, cyemi_105/1, cyemi_107/1
  cfblk12/1 -> cyemi_76/1, cyemi_101/1
  cfblk3/1 -> cyemi_88/1, cyemi_95/1, cyemi_96/1, cyemi_103/1, cyemi_108/1
  cfblk9/1 -> cyemi_90/1, cyemi_91/1
  cfblk6/1 -> cyemi_32/1, cyemi_99/1
  cfblk4/1 -> cfblk2/1
  cfblk10/1 -> cfblk14/Action
  cfblk10/2 -> cfblk15/Action
  cfblk11/1 -> cfblk16/Action
  cfblk11/2 -> cfblk17/Action
  cyemi_30/1 -> cfblk10/1
  cfblk23/1 -> cyemi_30/1
  cyemi_31/1 -> cfblk11/1
  cfblk1/1 -> cyemi_31/1
  cyemi_32/1 -> cfblk14/1(cfblk1)
  cyemi_37/1 -> cfblk15/1(cfblk1)
  cfblk24/1 -> cyemi_37/1
  cyemi_38/1 -> cfblk15/2(cfblk15)
  cfblk19/1 -> cyemi_38/1
  cyemi_39/1 -> cfblk15/3(cfblk16)
  cfblk14/1(cfblk2) -> cyemi_39/1
  cyemi_56/1 -> cfblk16/1(cfblk1)
  cfblk20/1 -> cyemi_56/1
  cyemi_57/1 -> cfblk16/2(cfblk11)
  cfblk28/1 -> cyemi_57/1
  cyemi_58/1 -> cfblk16/3(cfblk12)
  cfblk27/1 -> cyemi_58/1
  cyemi_59/1 -> cfblk16/4(cfblk13)
  cfblk29/1 -> cyemi_59/1
  cyemi_60/1 -> cfblk16/5(cfblk14)
  cfblk25/1 -> cyemi_60/1
  cyemi_73/1 -> cfblk17/1(cfblk1)
  cfblk18/1 -> cyemi_73/1
  cyemi_74/1 -> cfblk17/2(cfblk12)
  cfblk22/1 -> cyemi_74/1
  cyemi_75/1 -> cfblk17/3(cfblk13)
  cfblk21/1 -> cyemi_75/1
  cyemi_76/1 -> cfblk17/4(cfblk14)
  cyemi_77/1 -> cfblk17/5(cfblk15)
  cfblk26/1 -> cyemi_77/1
  cyemi_88/1 -> cfblk18/1
  cyemi_89/1 -> cfblk19/1
  cfblk17/1(cfblk2) -> cyemi_89/1
  cyemi_90/1 -> cfblk20/1
  cyemi_91/1 -> cfblk21/1
  cyemi_92/1 -> cfblk22/1
  cfblk7/1 -> cyemi_92/1
  cyemi_93/1 -> cfblk23/1
  cyemi_94/1 -> cfblk24/1
  cfblk8/1 -> cyemi_94/1
  cyemi_95/1 -> cfblk25/1
  cyemi_96/1 -> cfblk26/1
  cyemi_97/1 -> cfblk27/1
  cyemi_98/1 -> cfblk28/1
  cfblk14/2(cfblk7) -> cyemi_98/1
  cyemi_99/1 -> cfblk29/1
  cyemi_100/1 -> cfblk3/1
  cyemi_101/1 -> cfblk4/1
  cyemi_102/1 -> cfblk5/1
  cyemi_103/1 -> cfblk5/2
  cyemi_104/1 -> cfblk6/1
  cfblk16/1(cfblk2) -> cyemi_104/1
  cyemi_105/1 -> cfblk7/1
  cyemi_106/1 -> cfblk7/2
  cfblk13/1 -> cyemi_106/1
  cyemi_107/1 -> cfblk8/1
  cyemi_108/1 -> cfblk9/1

== system sampleModel7424_pp_difftest/cfblk125 ==
  cfblk1 : Inport
  cfblk9 : Inport  Port=2
  cfblk10 : Inport  Port=3
  Action Port : ActionPort  ActionType=then
  cfblk11 : Subsystem  TreatAsAtomicUnit=on
  cfblk12 : Subsystem  TreatAsAtomicUnit=on
  cfblk13 : Delay
  cfblk14 : Delay
  cfblk3 : simulink/Discrete/Transfer Fcn Real Zero  ZeroZ=0.75  ICPrevInput=0.0  DoSatur=off
      settings: SourceProductName=Simulink  SourceProductBaseCode=SL
  cfblk4 : Delay  DelayLengthSource=Input port
      settings: InputPortMap=u0,p1
  cfblk5 : simulink/Discrete/Transfer Fcn Lead or Lag  PoleZ=0.95  ZeroZ=0.75  ICPrevOutput=0.0  ICPrevInput=0.0  DoSatur=off
      settings: SourceProductName=Simulink  SourceProductBaseCode=SL
  cfblk6 : simulink/Discrete/Transfer Fcn Lead or Lag  PoleZ=0.95  ZeroZ=0.75  ICPrevOutput=0.0  ICPrevInput=0.0  DoSatur=off
      settings: SourceProductName=Simulink  SourceProductBaseCode=SL
  cfblk7 : DiscreteIntegrator  SampleTime=-1  OutDataTypeStr=double  ICPrevOutput=DiscIntNeverNeededParam  ICPrevScaledInput=DiscIntNeverNeededParam
  cfblk8 : If  SampleTime=1
  cyemi_{112..113,127,144..152} (12 alike) : DataTypeConversion  OutDataTypeStr=double
  cfblk2 : Outport
  wires:
  cfblk10/1 -> cfblk2/1
  cfblk8/1 -> cfblk11/Action
  cfblk8/2 -> cfblk12/Action
  cyemi_112/1 -> cfblk11/1(cfblk1)
  cfblk3/1 -> cyemi_112/1
  cyemi_113/1 -> cfblk11/2(cfblk12)
  cfblk12/1(cfblk2) -> cyemi_113/1
  cyemi_127/1 -> cfblk12/1(cfblk1)
  cfblk7/1 -> cyemi_127/1
  cyemi_144/1 -> cfblk13/1
  cfblk11/1(cfblk2) -> cyemi_144/1
  cyemi_145/1 -> cfblk14/1
  cfblk5/1 -> cyemi_145/1
  cyemi_146/1 -> cfblk3/1
  cfblk6/1 -> cyemi_146/1
  cyemi_147/1 -> cfblk4/1
  cfblk14/1 -> cyemi_147/1
  cyemi_148/1 -> cfblk4/2
  cfblk11/2(cfblk13) -> cyemi_148/1
  cyemi_149/1 -> cfblk5/1
  cfblk4/1 -> cyemi_149/1
  cyemi_150/1 -> cfblk6/1
  cfblk9/1 -> cyemi_150/1
  cyemi_151/1 -> cfblk7/1
  cfblk1/1 -> cyemi_151/1
  cyemi_152/1 -> cfblk8/1
  cfblk13/1 -> cyemi_152/1

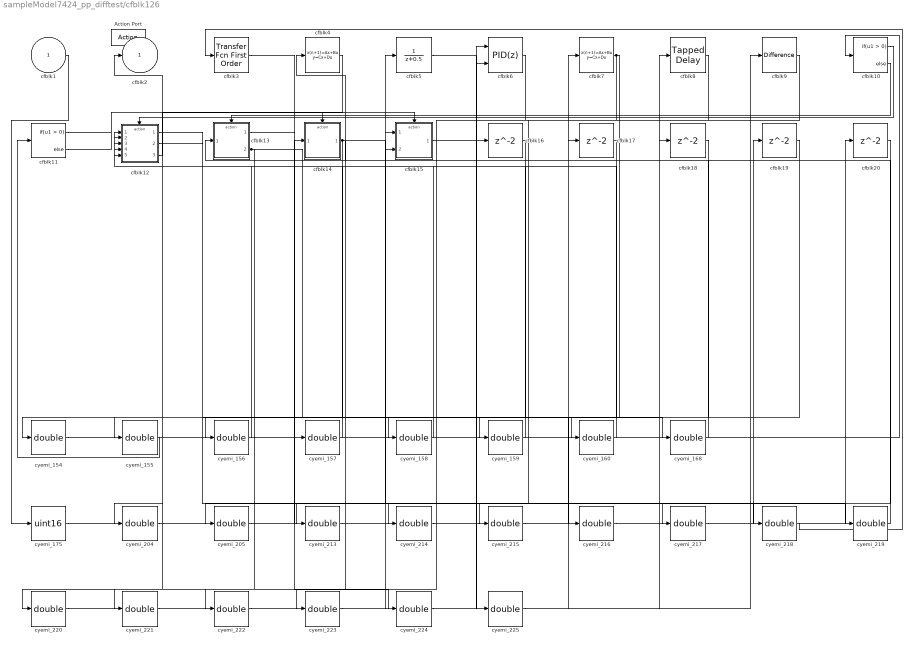
== system sampleModel7424_pp_difftest/cfblk126 ==
  cfblk1 : Inport
  Action Port : ActionPort  ActionType=else
  cfblk10 : If  SampleTime=1
  cfblk11 : If  SampleTime=1
  cfblk12 : Subsystem  TreatAsAtomicUnit=on
  cfblk13 : Subsystem  TreatAsAtomicUnit=on
  cfblk14 : Subsystem  TreatAsAtomicUnit=on
  cfblk15 : Subsystem  TreatAsAtomicUnit=on
  cfblk{16..20} (5 alike) : Delay
  cfblk3 : simulink/Discrete/Transfer Fcn First Order  PoleZ=0.95  ICPrevOutput=0.0  DoSatur=off
      settings: SourceProductName=Simulink
  cfblk4 : DiscreteStateSpace  SampleTime=-1
  cfblk5 : DiscreteTransferFcn
  cfblk6 : simulink/Continuous/PID Controller (2DOF)  Controller=PID  TimeDomain=Discrete-time  SampleTime=-1  IntegratorMethod=Forward Euler  FilterMethod=Forward Euler  Form=Parallel  UseFilter=on  ControllerParametersSource=internal  P=1  I=1  D=0  N=100  b=1  c=1  InitialConditionSource=internal  InitialConditionForIntegrator=0  InitialConditionForFilter=0  ExternalReset=none  LimitOutput=off  UpperSaturationLimit=inf  LowerSaturationLimit=-inf  LinearizeAsGain=off  AntiWindupMode=none  Kb=1  TrackingMode=off  Kt=1  PParamMin=[]  PParamMax=[]  IParamMin=[]  IParamMax=[]  DParamMin=[]  DParamMax=[]  NParamMin=[]  NParamMax=[]  bParamMin=[]  bParamMax=[]  cParamMin=[]  cParamMax=[]  KbParamMin=[]  KbParamMax=[]  KtParamMin=[]  KtParamMax=[]  POutMin=[]  POutMax=[]  IOutMin=[]  IOutMax=[]  DOutMin=[]  DOutMax=[]  NOutMin=[]  NOutMax=[]  bOutMin=[]  bOutMax=[]  cOutMin=[]  cOutMax=[]  KbOutMin=[]  KbOutMax=[]  KtOutMin=[]  KtOutMax=[]  IntegratorOutMin=[]  IntegratorOutMax=[]  FilterOutMin=[]  FilterOutMax=[]  SumOutMin=[]  SumOutMax=[]  Sum1OutMin=[]  Sum1OutMax=[]  Sum2OutMin=[]  Sum2OutMax=[]  Sum3OutMin=[]  Sum3OutMax=[]  SumI1OutMin=[]  SumI1OutMax=[]  SumI2OutMin=[]  SumI2OutMax=[]  SumI3OutMin=[]  SumI3OutMax=[]  SumDOutMin=[]  SumDOutMax=[]  SaturationOutMin=[]  SaturationOutMax=[]  IntegratorContinuousStateAttributes=''  IntegratorStateMustResolveToSignalObject=off  IntegratorRTWStateStorageClass=Auto  FilterContinuousStateAttributes=''  FilterStateMustResolveToSignalObject=off  FilterRTWStateStorageClass=Auto  DifferentiatorICPrevScaledInput=0  DifferentiatorOutMin=[]  DifferentiatorOutMax=[]  FilterDiffOutCoefMin=[]  FilterDiffOutCoefMax=[]  SumDenOutMin=[]  SumDenOutMax=[]  SumNumOutMin=[]  SumNumOutMax=[]  ReciprocalOutMin=[]  ReciprocalOutMax=[]  DivideOutMin=[]  DivideOutMax=[]  TunerSelectOption=Transfer Function Based (PID Tuner App)
  cfblk7 : DiscreteStateSpace  SampleTime=-1
  cfblk8 : simulink/Discrete/Tapped Delay  vinit=0.0  samptime=-1  NumDelays=1  DelayOrder=Oldest  includeCurrent=off
  cfblk9 : simulink/Discrete/Difference  ICPrevInput=0.0  OutMin=[]  OutMax=[]  OutDataTypeStr=double  OutputDataTypeScalingMode=double  OutDataType=fixdt(1, 16)  OutScaling=2^-10  DoSatur=off
  cyemi_{154..160,168,204..205,213..225} (23 alike) : DataTypeConversion  OutDataTypeStr=double
  cyemi_175 : DataTypeConversion  OutDataTypeStr=uint16
  cfblk2 : Outport
  wires:
  cfblk7/1 -> cyemi_156/1, cyemi_160/1, cyemi_220/1
  cfblk14/1(cfblk2) -> cyemi_154/1, cyemi_218/1, cyemi_223/1
  cfblk13/2(cfblk7) -> cyemi_216/1, cyemi_222/1
  cfblk12/3(cfblk15) -> cfblk2/1
  cfblk10/1 -> cfblk12/Action
  cfblk10/2 -> cfblk13/Action
  cfblk11/1 -> cfblk14/Action
  cfblk11/2 -> cfblk15/Action
  cyemi_154/1 -> cfblk10/1
  cyemi_155/1 -> cfblk11/1
  cfblk16/1 -> cyemi_155/1
  cyemi_156/1 -> cfblk12/1(cfblk1)
  cyemi_157/1 -> cfblk12/2(cfblk10)
  cfblk3/1 -> cyemi_157/1
  cyemi_158/1 -> cfblk12/3(cfblk11)
  cfblk18/1 -> cyemi_158/1
  cyemi_159/1 -> cfblk12/4(cfblk12)
  cfblk19/1 -> cyemi_159/1
  cyemi_160/1 -> cfblk12/5(cfblk13)
  cyemi_168/1 -> cfblk13/1(cfblk1)
  cfblk12/2(cfblk14) -> cyemi_168/1
  cyemi_175/1 -> cfblk14/1(cfblk1)
  cfblk1/1 -> cyemi_175/1
  cyemi_204/1 -> cfblk15/1(cfblk1)
  cfblk17/1 -> cyemi_204/1
  cyemi_205/1 -> cfblk15/2(cfblk9)
  cfblk20/1 -> cyemi_205/1
  cyemi_213/1 -> cfblk16/1
  cfblk6/1 -> cyemi_213/1
  cyemi_214/1 -> cfblk17/1
  cfblk9/1 -> cyemi_214/1
  cyemi_215/1 -> cfblk18/1
  cfblk8/1 -> cyemi_215/1
  cyemi_216/1 -> cfblk19/1
  cyemi_217/1 -> cfblk20/1
  cfblk5/1 -> cyemi_217/1
  cyemi_218/1 -> cfblk3/1
  cyemi_219/1 -> cfblk4/1
  cfblk12/1(cfblk2) -> cyemi_219/1
  cyemi_220/1 -> cfblk5/1
  cyemi_221/1 -> cfblk6/1
  cfblk4/1 -> cyemi_221/1
  cyemi_222/1 -> cfblk6/2
  cyemi_223/1 -> cfblk7/1
  cyemi_224/1 -> cfblk8/1
  cfblk13/1(cfblk2) -> cyemi_224/1
  cyemi_225/1 -> cfblk9/1
  cfblk15/1(cfblk2) -> cyemi_225/1

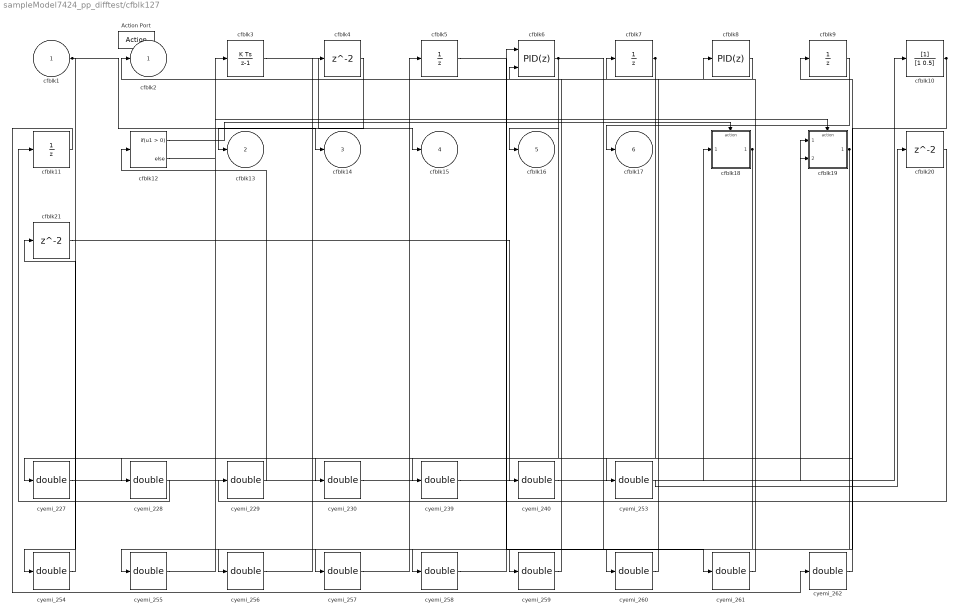
== system sampleModel7424_pp_difftest/cfblk127 ==
  cfblk1 : Inport
  Action Port : ActionPort  ActionType=then
  cfblk10 : DiscreteFilter
  cfblk{5,7,9,11} (4 alike) : UnitDelay  SampleTime=-1
  cfblk12 : If  SampleTime=1
  cfblk18 : Subsystem  TreatAsAtomicUnit=on
  cfblk19 : Subsystem  TreatAsAtomicUnit=on
  cfblk20 : Delay
  cfblk21 : Delay
  cfblk3 : DiscreteIntegrator  SampleTime=-1  OutDataTypeStr=double  ICPrevOutput=DiscIntNeverNeededParam  ICPrevScaledInput=DiscIntNeverNeededParam
  cfblk4 : Delay
  cfblk6 : simulink/Continuous/PID Controller (2DOF)  Controller=PID  TimeDomain=Discrete-time  SampleTime=-1  IntegratorMethod=Forward Euler  FilterMethod=Forward Euler  Form=Parallel  UseFilter=on  ControllerParametersSource=internal  P=1  I=1  D=0  N=100  b=1  c=1  InitialConditionSource=internal  InitialConditionForIntegrator=0  InitialConditionForFilter=0  ExternalReset=none  LimitOutput=off  UpperSaturationLimit=inf  LowerSaturationLimit=-inf  LinearizeAsGain=off  AntiWindupMode=none  Kb=1  TrackingMode=off  Kt=1  PParamMin=[]  PParamMax=[]  IParamMin=[]  IParamMax=[]  DParamMin=[]  DParamMax=[]  NParamMin=[]  NParamMax=[]  bParamMin=[]  bParamMax=[]  cParamMin=[]  cParamMax=[]  KbParamMin=[]  KbParamMax=[]  KtParamMin=[]  KtParamMax=[]  POutMin=[]  POutMax=[]  IOutMin=[]  IOutMax=[]  DOutMin=[]  DOutMax=[]  NOutMin=[]  NOutMax=[]  bOutMin=[]  bOutMax=[]  cOutMin=[]  cOutMax=[]  KbOutMin=[]  KbOutMax=[]  KtOutMin=[]  KtOutMax=[]  IntegratorOutMin=[]  IntegratorOutMax=[]  FilterOutMin=[]  FilterOutMax=[]  SumOutMin=[]  SumOutMax=[]  Sum1OutMin=[]  Sum1OutMax=[]  Sum2OutMin=[]  Sum2OutMax=[]  Sum3OutMin=[]  Sum3OutMax=[]  SumI1OutMin=[]  SumI1OutMax=[]  SumI2OutMin=[]  SumI2OutMax=[]  SumI3OutMin=[]  SumI3OutMax=[]  SumDOutMin=[]  SumDOutMax=[]  SaturationOutMin=[]  SaturationOutMax=[]  IntegratorContinuousStateAttributes=''  IntegratorStateMustResolveToSignalObject=off  IntegratorRTWStateStorageClass=Auto  FilterContinuousStateAttributes=''  FilterStateMustResolveToSignalObject=off  FilterRTWStateStorageClass=Auto  DifferentiatorICPrevScaledInput=0  DifferentiatorOutMin=[]  DifferentiatorOutMax=[]  FilterDiffOutCoefMin=[]  FilterDiffOutCoefMax=[]  SumDenOutMin=[]  SumDenOutMax=[]  SumNumOutMin=[]  SumNumOutMax=[]  ReciprocalOutMin=[]  ReciprocalOutMax=[]  DivideOutMin=[]  DivideOutMax=[]  TunerSelectOption=Transfer Function Based (PID Tuner App)
  cfblk8 : simulink/Continuous/PID Controller  Controller=PID  TimeDomain=Discrete-time  SampleTime=-1  IntegratorMethod=Forward Euler  FilterMethod=Forward Euler  Form=Parallel  UseFilter=on  ControllerParametersSource=internal  P=1  I=1  D=0  N=100  InitialConditionSource=internal  InitialConditionForIntegrator=0  InitialConditionForFilter=0  ExternalReset=none  LimitOutput=off  UpperSaturationLimit=inf  LowerSaturationLimit=-inf  LinearizeAsGain=off  AntiWindupMode=none  Kb=1  TrackingMode=off  Kt=1  PParamMin=[]  PParamMax=[]  IParamMin=[]  IParamMax=[]  DParamMin=[]  DParamMax=[]  NParamMin=[]  NParamMax=[]  KbParamMin=[]  KbParamMax=[]  KtParamMin=[]  KtParamMax=[]  POutMin=[]  POutMax=[]  IOutMin=[]  IOutMax=[]  DOutMin=[]  DOutMax=[]  NOutMin=[]  NOutMax=[]  KbOutMin=[]  KbOutMax=[]  KtOutMin=[]  KtOutMax=[]  IntegratorOutMin=[]  IntegratorOutMax=[]  FilterOutMin=[]  FilterOutMax=[]  SumOutMin=[]  SumOutMax=[]  SumI1OutMin=[]  SumI1OutMax=[]  SumI2OutMin=[]  SumI2OutMax=[]  SumI3OutMin=[]  SumI3OutMax=[]  SumDOutMin=[]  SumDOutMax=[]  SaturationOutMin=[]  SaturationOutMax=[]  IntegratorContinuousStateAttributes=''  IntegratorStateMustResolveToSignalObject=off  IntegratorRTWStateStorageClass=Auto  FilterContinuousStateAttributes=''  FilterStateMustResolveToSignalObject=off  FilterRTWStateStorageClass=Auto  DifferentiatorICPrevScaledInput=0  DifferentiatorOutMin=[]  DifferentiatorOutMax=[]  FilterDiffOutCoefMin=[]  FilterDiffOutCoefMax=[]  SumDenOutMin=[]  SumDenOutMax=[]  SumNumOutMin=[]  SumNumOutMax=[]  ReciprocalOutMin=[]  ReciprocalOutMax=[]  DivideOutMin=[]  DivideOutMax=[]  TunerSelectOption=Transfer Function Based (PID Tuner App)
  cyemi_{227..230,239..240,253..262} (16 alike) : DataTypeConversion  OutDataTypeStr=double
  cfblk2 : Outport
  cfblk13 : Outport  Port=2
  cfblk14 : Outport  Port=3
  cfblk15 : Outport  Port=4
  cfblk16 : Outport  Port=5
  cfblk17 : Outport  Port=6
  wires:
  cfblk9/1 -> cfblk17/1
  cfblk8/1 -> cfblk2/1
  cfblk7/1 -> cyemi_253/1, cyemi_254/1
  cfblk19/1(cfblk2) -> cyemi_228/1, cyemi_257/1
  cfblk18/1(cfblk2) -> cyemi_255/1, cyemi_256/1
  cfblk10/1 -> cyemi_230/1, cyemi_258/1, cyemi_259/1
  cfblk6/1 -> cfblk16/1, cyemi_239/1, cyemi_261/1
  cfblk4/1 -> cfblk13/1
  cfblk1/1 -> cfblk14/1, cyemi_227/1
  cfblk3/1 -> cfblk15/1
  cfblk12/1 -> cfblk18/Action
  cfblk12/2 -> cfblk19/Action
  cyemi_227/1 -> cfblk10/1
  cyemi_228/1 -> cfblk11/1
  cyemi_229/1 -> cfblk12/1
  cfblk20/1 -> cyemi_229/1
  cyemi_230/1 -> cfblk18/1(cfblk1)
  cyemi_239/1 -> cfblk19/1(cfblk1)
  cyemi_240/1 -> cfblk19/2(cfblk10)
  cfblk21/1 -> cyemi_240/1
  cyemi_253/1 -> cfblk20/1
  cyemi_254/1 -> cfblk21/1
  cyemi_255/1 -> cfblk3/1
  cyemi_256/1 -> cfblk4/1
  cyemi_257/1 -> cfblk5/1
  cyemi_258/1 -> cfblk6/1
  cyemi_259/1 -> cfblk6/2
  cyemi_260/1 -> cfblk7/1
  cfblk5/1 -> cyemi_260/1
  cyemi_261/1 -> cfblk8/1
  cyemi_262/1 -> cfblk9/1
  cfblk11/1 -> cyemi_262/1

== system sampleModel7424_pp_difftest/cfblk128 ==
  cfblk1 : Inport
  cfblk9 : Inport  Port=2
  cfblk10 : Inport  Port=3
  Action Port : ActionPort  ActionType=else
  cfblk13 : DataTypeConversion  OutDataTypeStr=double
  cfblk14 : DataTypeConversion  OutDataTypeStr=double
  cfblk3 : simulink/Discrete/Transfer Fcn Lead or Lag  PoleZ=0.95  ZeroZ=0.75  ICPrevOutput=0.0  ICPrevInput=0.0  DoSatur=off
      settings: SourceProductName=Simulink  SourceProductBaseCode=SL
  cfblk4 : DiscreteIntegrator  SampleTime=-1  OutDataTypeStr=double  ICPrevOutput=DiscIntNeverNeededParam  ICPrevScaledInput=DiscIntNeverNeededParam
  cfblk5 : UnitDelay  SampleTime=-1
  cfblk6 : simulink/Discrete/Transfer Fcn First Order  PoleZ=0.95  ICPrevOutput=0.0  DoSatur=off
      settings: SourceProductName=Simulink
  cfblk7 : DiscreteStateSpace  SampleTime=-1
  cfblk8 : simulink/Discrete/Transfer Fcn Real Zero  ZeroZ=0.75  ICPrevInput=0.0  DoSatur=off
      settings: SourceProductName=Simulink  SourceProductBaseCode=SL
  cyemi_{266,269..270,272} (4 alike) : DataTypeConversion  OutDataTypeStr=double
  cyemi_267 : DataTypeConversion  OutDataTypeStr=fixdt('ufix16_E3')
  cyemi_268 : DataTypeConversion  OutDataTypeStr=uint16
  cyemi_271 : DataTypeConversion  OutDataTypeStr=fixdt('ufix16_E3')
  cyemi_273 : DataTypeConversion  OutDataTypeStr=fixdt('ufix16_E3')
  cfblk2 : Outport
  cfblk11 : Outport  Port=2
  cfblk12 : Outport  Port=3
  wires:
  cfblk5/1 -> cfblk11/1
  cfblk7/1 -> cfblk12/1
  cfblk10/1 -> cfblk2/1
  cyemi_266/1 -> cfblk13/1
  cfblk4/1 -> cyemi_266/1
  cyemi_267/1 -> cfblk14/1
  cfblk6/1 -> cyemi_267/1
  cyemi_268/1 -> cfblk3/1
  cfblk1/1 -> cyemi_268/1
  cyemi_269/1 -> cfblk4/1
  cfblk14/1 -> cyemi_269/1
  cyemi_270/1 -> cfblk5/1
  cfblk9/1 -> cyemi_270/1
  cyemi_271/1 -> cfblk6/1
  cfblk8/1 -> cyemi_271/1
  cyemi_272/1 -> cfblk7/1
  cfblk13/1 -> cyemi_272/1
  cyemi_273/1 -> cfblk8/1
  cfblk3/1 -> cyemi_273/1
